simulink library "imu_library"  (R2019b)
settings: Solver=VariableStepAuto  StartTime=0.0  StopTime=10.0  RelTol=1e-3
values from neighbouring files (symbols this model uses):
  g = 9.81    [robotParameters.m]
  imu_sample_rate = 100    [robotParameters.m]
libraries: nesl_utility x7, simulink x6, sm_lib x1, aerolibutil x1
settings Model: Creator=vuwij  LastModifiedBy=vuwij

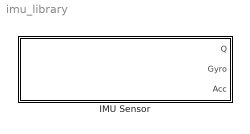
== system imu_library ==
  IMU Sensor : Subsystem

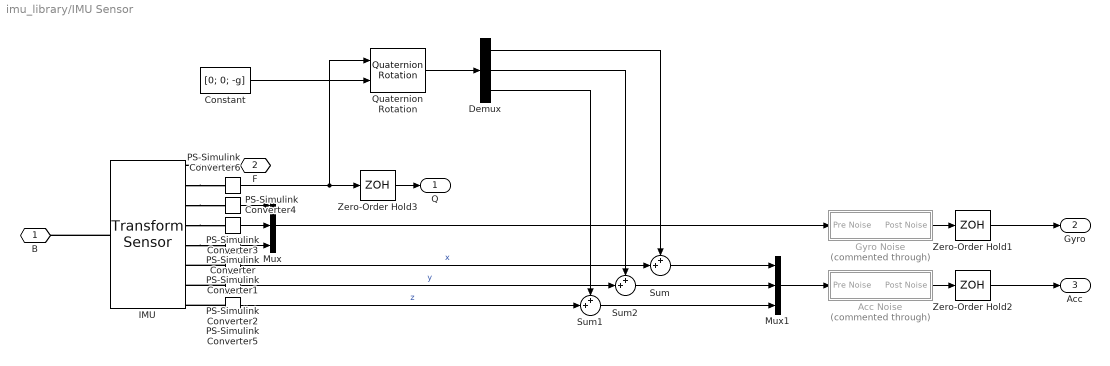
== system imu_library/IMU Sensor ==
  Acc Noise : Subsystem  Commented=through
  Constant : Constant  Value=[0; 0; -g]
  Demux : Demux  Outputs=3
  Gyro Noise : Subsystem  Commented=through
  IMU : sm_lib/Frames and Transforms/Transform Sensor  MeasurementFrame=Follower  SenseAngle=off  SenseAxis=off  SenseAngle1=off  SenseAngle2=off  SenseAngle3=off  SenseQ=on  SenseR=off  SenseOmegaX=on  SenseOmegaY=on  SenseOmegaZ=on  SenseOmega1=off  SenseOmega2=off  SenseOmega3=off  SenseQDot=off  SenseRDot=off  SenseAlphaX=off  SenseAlphaY=off  SenseAlphaZ=off  SenseAlpha1=off  SenseAlpha2=off  SenseAlpha3=off  SenseQDDot=off  SenseRDDot=off  SenseX=off  SenseY=off  SenseZ=off  SenseRad=off  SenseAzim=off  SenseDist=off  SenseInc=off  SenseXDot=off  SenseYDot=off  SenseZDot=off  SenseRadDot=off  SenseAzimDot=off  SenseDistDot=off  SenseIncDot=off  SenseXDDot=on  SenseYDDot=on  SenseZDDot=on  SenseRadDDot=off  SenseAzimDDot=off  SenseDistDDot=off  SenseIncDDot=off
  Mux : Mux  Inputs=3
  Mux1 : Mux  Inputs=3
  PS-Simulink Converter{,1..6} (7 alike) : nesl_utility/PS-Simulink Converter  PhysicalDomain=network_engine_domain  SubClassName=ps_output  LeftPortType=input  RightPortType=output  PseudoPeriodic=off  Frequencies=[]  Unit=inherit  AffineConversion=off
  Quaternion Rotation : aerolibutil/Quaternion Rotation
  Sum : Sum  Inputs=++|
  Sum1 : Sum  Inputs=++|
  Sum2 : Sum  Inputs=++|
  Zero-Order Hold1 : ZeroOrderHold  SampleTime=1/imu_sample_rate
  Zero-Order Hold2 : ZeroOrderHold  SampleTime=1/imu_sample_rate
  Zero-Order Hold3 : ZeroOrderHold  SampleTime=1/imu_sample_rate
  B : PMIOPort  Side=Left
  F : PMIOPort  Port=2  Side=Left
  Q : Outport
  Gyro : Outport  Port=2
  Acc : Outport  Port=3
  wires:
  Mux1/1 -> Acc Noise/1(Pre Noise)
  Zero-Order Hold2/1 -> Acc/1
  PS-Simulink Converter2/1 -> Sum2/2  "y"
  Demux/3 -> Sum1/1
  Sum2/1 -> Mux1/2
  Demux/1 -> Sum/1
  Zero-Order Hold1/1 -> Gyro/1
  Gyro Noise/1(Post Noise) -> Zero-Order Hold1/1
  Acc Noise/1(Post Noise) -> Zero-Order Hold2/1
  PS-Simulink Converter1/1 -> Sum/2  "x"
  PS-Simulink Converter4/1 -> Mux/1
  Sum1/1 -> Mux1/3
  PS-Simulink Converter3/1 -> Mux/2
  Mux/1 -> Gyro Noise/1(Pre Noise)
  PS-Simulink Converter/1 -> Mux/3
  PS-Simulink Converter5/1 -> Sum1/2  "z"
  Constant/1 -> Quaternion Rotation/2
  PS-Simulink Converter6/1 -> Quaternion Rotation/1, Zero-Order Hold3/1
  Quaternion Rotation/1 -> Demux/1
  Sum/1 -> Mux1/1
  Demux/2 -> Sum2/1
  Zero-Order Hold3/1 -> Q/1
  connections:
  IMU/RConn2 -- PS-Simulink Converter6/LConn1
  IMU/LConn1 -- B/RConn1
  F/RConn1 -- IMU/RConn1
  PS-Simulink Converter1/LConn1 -- IMU/RConn6
  PS-Simulink Converter2/LConn1 -- IMU/RConn7
  PS-Simulink Converter5/LConn1 -- IMU/RConn8
  IMU/RConn5 -- PS-Simulink Converter/LConn1
  IMU/RConn4 -- PS-Simulink Converter3/LConn1
  IMU/RConn3 -- PS-Simulink Converter4/LConn1

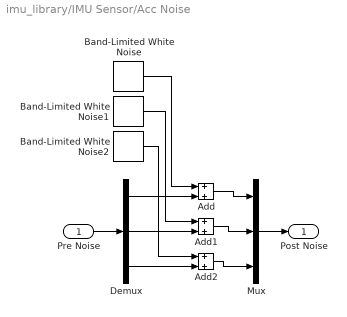
== system imu_library/IMU Sensor/Acc Noise ==
  Pre Noise : Inport
  Add : Sum  Inputs=2
  Add1 : Sum  Inputs=2
  Add2 : Sum  Inputs=2
  Band-Limited White Noise : simulink/Sources/Band-Limited White Noise  Cov=acc_noise  Ts=1/imu_sample_rate  seed=[21341]
  Band-Limited White Noise1 : simulink/Sources/Band-Limited White Noise  Cov=acc_noise  Ts=1/imu_sample_rate  seed=[13333]
  Band-Limited White Noise2 : simulink/Sources/Band-Limited White Noise  Cov=acc_noise  Ts=1/imu_sample_rate  seed=[13221]
  Demux : Demux  Outputs=3
  Mux : Mux  Inputs=3
  Post Noise : Outport
  wires:
  Mux/1 -> Post Noise/1
  Add2/1 -> Mux/3
  Add1/1 -> Mux/2
  Band-Limited White Noise2/1 -> Add2/1
  Band-Limited White Noise1/1 -> Add1/1
  Band-Limited White Noise/1 -> Add/1
  Pre Noise/1 -> Demux/1
  Add/1 -> Mux/1
  Demux/1 -> Add/2
  Demux/2 -> Add1/2
  Demux/3 -> Add2/2

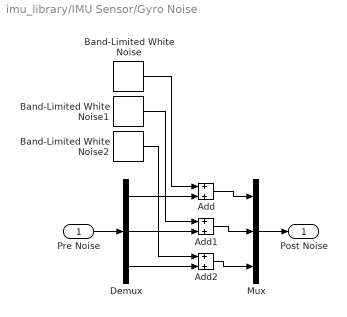
== system imu_library/IMU Sensor/Gyro Noise ==
  Pre Noise : Inport
  Add : Sum  Inputs=2
  Add1 : Sum  Inputs=2
  Add2 : Sum  Inputs=2
  Band-Limited White Noise : simulink/Sources/Band-Limited White Noise  Cov=gyro_noise  Ts=1/imu_sample_rate  seed=[23341]
  Band-Limited White Noise1 : simulink/Sources/Band-Limited White Noise  Cov=gyro_noise  Ts=1/imu_sample_rate  seed=[23333]
  Band-Limited White Noise2 : simulink/Sources/Band-Limited White Noise  Cov=gyro_noise  Ts=1/imu_sample_rate  seed=[13341]
  Demux : Demux  Outputs=3
  Mux : Mux  Inputs=3
  Post Noise : Outport
  wires:
  Mux/1 -> Post Noise/1
  Add2/1 -> Mux/3
  Add1/1 -> Mux/2
  Band-Limited White Noise2/1 -> Add2/1
  Band-Limited White Noise1/1 -> Add1/1
  Band-Limited White Noise/1 -> Add/1
  Pre Noise/1 -> Demux/1
  Add/1 -> Mux/1
  Demux/1 -> Add/2
  Demux/2 -> Add1/2
  Demux/3 -> Add2/2
